simulink model "Qi_4D"  (R2014b)
settings: Solver=ode45  StartTime=0.0  StopTime=10.0  RelTol=1e-3
values from neighbouring files (symbols this model uses):
  a = 0.95    [Run_Aizawa.m]    (also in Run_Arneodo.m = -5.5; Run_Chen.m = 33; Run_Chua.m = 15.6; Run_Chua_4D.m = 0.03)
  b = 0.7    [Run_Aizawa.m]    (also in Run_Arneodo.m = 3.5; Run_Chen.m = 3; Run_Chua.m = 28; Run_Duffing.m = 100)
  c = -1    [Run_Arneodo.m]    (also in Run_Chen.m = 25; Run_Chua_4D.m = -1.2; Run_Dadras.m = 2; Run_HindmarshRose.m = 1)
  d = 4 * 1e-3    (= 0.004)    [Run_Belousov_Zhabotinsky.m]    (also in Run_HindmarshRose.m = 5; Run_Qi_4D.m = 0.6; Run_Roessler_4D.m = 0.05)
undefined symbols (not defined in the file or in its folder): param
settings Model: Creator=Arek  LastModifiedBy=Arek

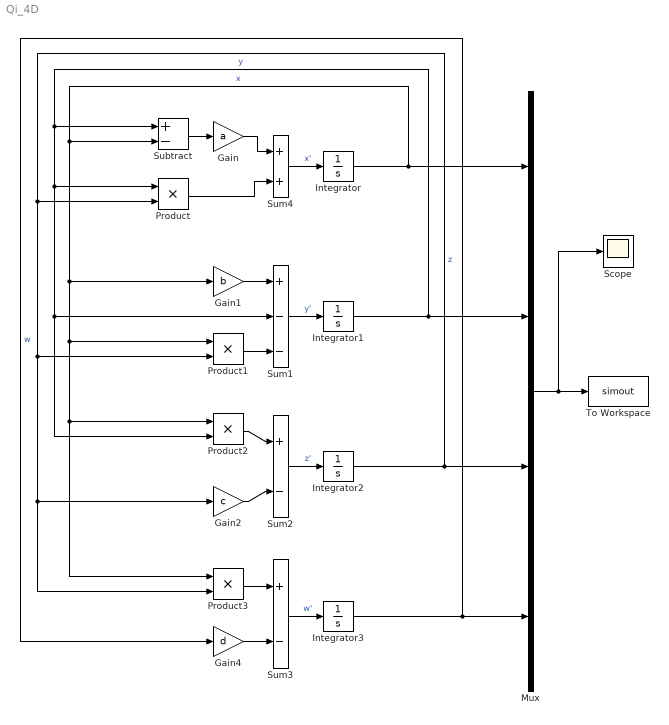
== system Qi_4D ==
  Gain : Gain  Gain=a
  Gain1 : Gain  Gain=b
  Gain2 : Gain  Gain=c
  Gain4 : Gain  Gain=d
  Integrator : Integrator  InitialCondition=param.ic(1)
  Integrator1 : Integrator  InitialCondition=param.ic(2)
  Integrator2 : Integrator  InitialCondition=param.ic(3)
  Integrator3 : Integrator  InitialCondition=param.ic(4)
  Mux : Mux
  Product{,1..3} (4 alike) : Product
  Scope : Scope
      settings: ShowLegends=on  TimeRange=0.05  YMin=-6  YMax=2
  Subtract : Sum  Inputs=+-
  Sum1 : Sum  Inputs=+--
  Sum2 : Sum  Inputs=+|-
  Sum3 : Sum  Inputs=+-
  Sum4 : Sum
  To Workspace : ToWorkspace  VariableName=simout  SaveFormat=Timeseries  SampleTime=-1
  wires:
  Sum2/1 -> Integrator2/1  "z'"
  Sum1/1 -> Integrator1/1  "y'"
  Sum4/1 -> Integrator/1  "x'"
  Integrator/1 -> Subtract/2, Gain1/1, Product1/1, Product3/1, Product2/1, Mux/1  "x"
  Integrator1/1 -> Subtract/1, Product2/2, Sum1/2, Product/1, Mux/2  "y"
  Integrator2/1 -> Product3/2, Gain2/1, Product1/2, Product/2, Mux/3  "z"
  Mux/1 -> Scope/1, To Workspace/1
  Integrator3/1 -> Gain4/1, Mux/4  "w"
  Gain4/1 -> Sum3/2
  Sum3/1 -> Integrator3/1  "w'"
  Subtract/1 -> Gain/1
  Gain/1 -> Sum4/1
  Product/1 -> Sum4/2
  Gain1/1 -> Sum1/1
  Product1/1 -> Sum1/3
  Product2/1 -> Sum2/1
  Gain2/1 -> Sum2/2
  Product3/1 -> Sum3/1
